simulink model "MoPhongRBKC"  (R2016a)
settings: Solver=VariableStepAuto  StartTime=0.0  StopTime=160  RelTol=1e-3
libraries: mblibv1 x18, simulink x3
settings Model: Creator=Nguyen Nam  LastModifiedBy=nguye
settings OptimizationCC: BlockReduction=off
settings GRTTargetCC: GeneratePreprocessorConditionals=Use local settings
settings SimMechanicsCC: VisOnUpdateDiagram=on  VisDuringSimulation=on

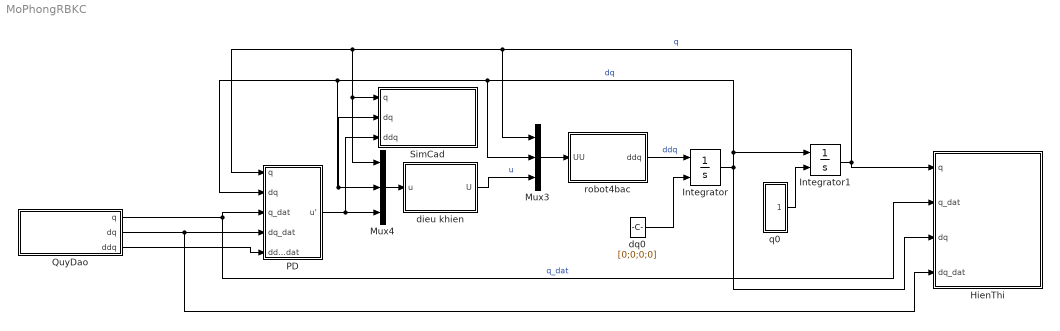
== system MoPhongRBKC ==
  HienThi : Subsystem  TreatAsAtomicUnit=on
  Integrator : Integrator  InitialConditionSource=external
  Integrator1 : Integrator  InitialConditionSource=external
  Mux3 : Mux  Inputs=3
  Mux4 : Mux  Inputs=3
  "PD " : Subsystem
  QuyDao : Subsystem  TreatAsAtomicUnit=on
  SimCad : Subsystem  TreatAsAtomicUnit=on
  dieu khien : MATLAB Function  TreatAsAtomicUnit=on
  dq0 : Constant  Value=[0;0;0;0]
  q0 : Subsystem
  robot4bac : MATLAB Function  TreatAsAtomicUnit=on
  wires:
  QuyDao/1(q) -> HienThi/2(q_dat), "PD "/3(q_dat)  "q_dat"
  Mux3/1 -> robot4bac/1(UU)
  robot4bac/1(ddq) -> Integrator/1  "ddq"
  Integrator/1 -> HienThi/3(dq), "PD "/2(dq), Mux4/2, SimCad/2(dq), Mux3/2, Integrator1/1  "dq"
  Integrator1/1 -> "PD "/1(q), Mux4/1, SimCad/1(q), Mux3/1, HienThi/1(q)  "q"
  q0/1("q0 ") -> Integrator1/2
  dq0/1 -> Integrator/2
  Mux4/1 -> dieu khien/1(u)
  "PD "/1(u') -> SimCad/3(ddq), Mux4/3
  dieu khien/1(U) -> Mux3/3  "u"
  QuyDao/3(ddq) -> "PD "/5(ddq_dat)
  QuyDao/2(dq) -> HienThi/4(dq_dat), "PD "/4(dq_dat)

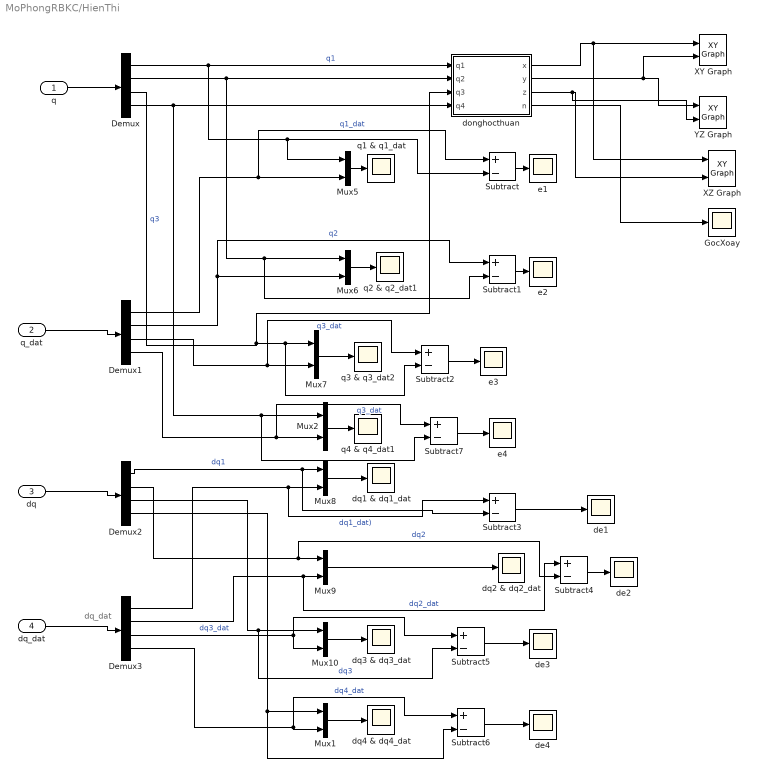
== system MoPhongRBKC/HienThi ==
  note: dq_dat
  q : Inport
  q_dat : Inport  Port=2
  dq : Inport  Port=3
  dq_dat : Inport  Port=4
  Demux{,1..3} (4 alike) : Demux
  GocXoay : Scope
  Mux{1..2,5..10} (8 alike) : Mux  Inputs=2
  Subtract{,1..7} (8 alike) : Sum  Inputs=+-
  XY Graph : simulink/Sinks/XY Graph  xmin=-10  xmax=500  ymin=-10  ymax=300  st=0
  XZ Graph : simulink/Sinks/XY Graph  xmin=-100  xmax=500  ymin=-100  ymax=300  st=0
  YZ Graph : simulink/Sinks/XY Graph  xmin=-100  xmax=300  ymin=-100  ymax=300  st=0
  de{1..4} (4 alike) : Scope
  donghocthuan : MATLAB Function  TreatAsAtomicUnit=on
  dq1 & dq1_dat : Scope
  dq2 & dq2_dat : Scope
  dq3 & dq3_dat : Scope
  dq4 & dq4_dat : Scope
  e{1..4} (4 alike) : Scope
  q1 & q1_dat : Scope
  q2 & q2_dat1 : Scope
  q3 & q3_dat2 : Scope
  q4 & q4_dat1 : Scope
  wires:
  q/1 -> Demux/1
  Demux/1 -> Subtract/2, Mux5/1, donghocthuan/1(q1)  "q1"
  Mux5/1 -> q1 & q1_dat/1
  Demux/2 -> Subtract1/2, Mux6/1, donghocthuan/2(q2)
  Demux1/2 -> Mux6/2, Subtract1/1  "q2"
  Demux1/3 -> Subtract2/1, Mux7/2  "q3_dat"
  Mux6/1 -> q2 & q2_dat1/1
  Demux2/1 -> Subtract3/2, Mux8/1  "dq1"
  Demux3/1 -> Subtract3/1, Mux8/2  "dq1_dat)"
  Mux8/1 -> dq1 & dq1_dat/1
  Demux2/2 -> Subtract4/2, Mux9/1  "dq2"
  Demux3/2 -> Subtract4/1, Mux9/2  "dq2_dat"
  Demux3/3 -> Mux10/2, Subtract5/1  "dq3_dat"
  Demux2/3 -> Subtract5/2, Mux10/1  "dq3"
  Mux10/1 -> dq3 & dq3_dat/1
  Mux9/1 -> dq2 & dq2_dat/1
  Mux7/1 -> q3 & q3_dat2/1
  Demux1/1 -> Subtract/1, Mux5/2  "q1_dat"
  donghocthuan/1(x) -> XZ Graph/1, XY Graph/1
  donghocthuan/2(y) -> YZ Graph/1, XY Graph/2
  Subtract/1 -> e1/1
  Subtract1/1 -> e2/1
  Subtract2/1 -> e3/1
  Subtract3/1 -> de1/1
  Subtract4/1 -> de2/1
  Subtract5/1 -> de3/1
  q_dat/1 -> Demux1/1
  dq/1 -> Demux2/1
  dq_dat/1 -> Demux3/1
  donghocthuan/4(n) -> GocXoay/1
  Demux/4 -> Subtract7/2, Mux2/1, donghocthuan/4(q4)
  Demux3/4 -> Mux1/2, Subtract6/1  "dq4_dat"
  Demux2/4 -> Subtract6/2, Mux1/1
  Mux1/1 -> dq4 & dq4_dat/1
  Subtract6/1 -> de4/1
  Demux1/4 -> Subtract7/1, Mux2/2  "q3_dat"
  Demux/3 -> donghocthuan/3(q3), Subtract2/2, Mux7/1  "q3"
  Mux2/1 -> q4 & q4_dat1/1
  Subtract7/1 -> e4/1
  donghocthuan/3(z) -> YZ Graph/2, XZ Graph/2

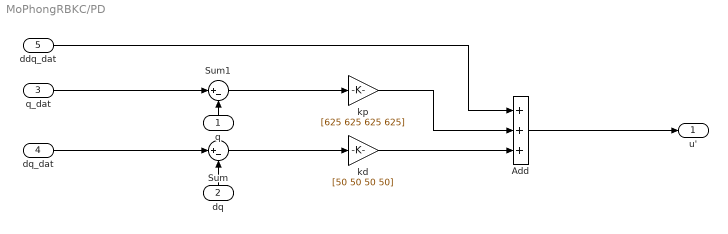
== system MoPhongRBKC/PD  ==
  q : Inport
  dq : Inport  Port=2
  q_dat : Inport  Port=3
  dq_dat : Inport  Port=4
  ddq_dat : Inport  Port=5
  Add : Sum  Inputs=3
  Sum : Sum  Inputs=|+-
  Sum1 : Sum  Inputs=|+-
  kd : Gain  Gain=[50 50 50 50]
  kp : Gain  Gain=[625 625 625 625]
  u' : Outport
  wires:
  Sum1/1 -> kp/1
  Sum/1 -> kd/1
  Add/1 -> u'/1
  ddq_dat/1 -> Add/1
  dq_dat/1 -> Sum/1
  q_dat/1 -> Sum1/1
  dq/1 -> Sum/2
  q/1 -> Sum1/2
  kd/1 -> Add/3
  kp/1 -> Add/2

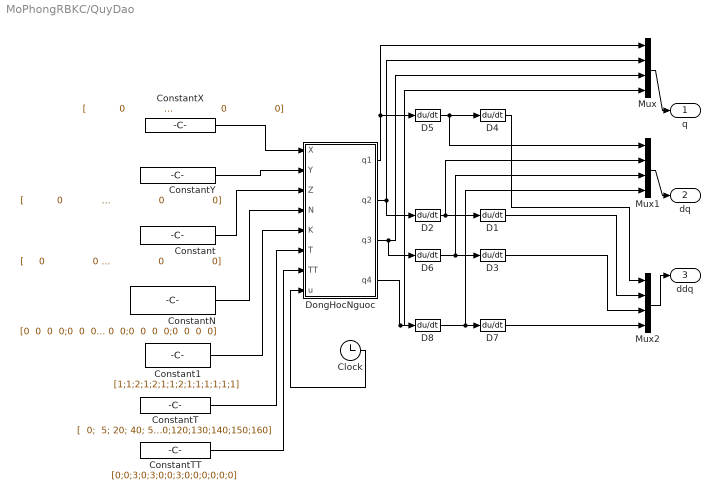
== system MoPhongRBKC/QuyDao ==
  Clock : Clock
      settings: Decimation=600
  Constant : Constant  Value="[     0                0               -6              0.8                0                0;   -50                0                0                0                0                0;   -50                0                0                0              -50                0;   -50                0                0                0                0                0;   -50                0                0                0              -50                0;   -50                0                0                0                0                0;   -50                0                0                0                0                0;   -50                0                0                0              -50                0;   -50                0                0                0                0                0;   -50                0                0                0                0                0;   -50                0                0                0                0                0;   -50                0                0                0                0                0;   -50                0                0                0                0                0;371200            -7200             46.5             -0.1                0                0]"
  Constant1 : Constant  Value=[1;1;2;1;2;1;1;2;1;1;1;1;1;1]
  ConstantN : Constant  Value="[0  0  0  0;0  0  0  0;0  0  0  0;0  0  0  0;0  0  0  0;0  0  0  0;0  0  0  0;0  0  0  0;0  0  0  0;0  0  0  0;0  0  0  0;0  0  0  0;0  0  0  0;0  0  0  0]"
  ConstantT : Constant  Value="[  0;  5; 20; 40; 50; 70; 80; 90;100;110;120;130;140;150;160]"
  ConstantTT : Constant  Value=[0;0;3;0;3;0;0;3;0;0;0;0;0;0]
  ConstantX : Constant  Value="[           0                0                0                0                0                0; 15.27777778     -6.666666667     0.8333333333   -0.02222222222                0                0; 14.13716694     -1.884955592    0.07068583471 -0.0007853981634               75             37.5;     31792.5            -2160             48.6            -0.36                0                0; 155.5088364     -8.246680716     0.1413716694 -0.0007853981634              330             37.5;       27440            -1092           14.625           -0.065                0                0;         400                0                0                0                0                0;-2670.353756      84.82300165    -0.8953539063   0.003141592654              390               10;     -229610             6600              -63              0.2                0                0;      -90460             2376            -20.7             0.06                0                0;     -621820            14976             -120             0.32                0                0;     -490000            10920              -81              0.2                0                0;           0                0                0                0                0                0;           0                0                0                0                0                0]"
  ConstantY : Constant  Value="[           0                0                0                0                0                0;           0                0                0                0                0                0; 14.13716694     -1.884955592    0.07068583471 -0.0007853981634                0             37.5;           0                0                0                0                0                0; 155.5088364     -8.246680716     0.1413716694 -0.0007853981634                0             37.5;           0                0                0                0                0                0;       85120            -3024             35.7            -0.14                0                0;-2670.353756      84.82300165    -0.8953539063   0.003141592654               70               10;          80                0                0                0                0                0;      121080            -3168             27.6            -0.08                0                0;         120                0                0                0                0                0;     -269435             6006           -44.55             0.11                0                0;     -394875             8190           -56.55             0.13                0                0;           0                0                0                0                0                0]"
  D{1..8} (8 alike) : Derivative
  DongHocNguoc : MATLAB Function  TreatAsAtomicUnit=on
  Mux : Mux
  Mux1 : Mux
  Mux2 : Mux
  q : Outport
  dq : Outport  Port=2
  ddq : Outport  Port=3
  wires:
  ConstantT/1 -> DongHocNguoc/6(T)
  ConstantY/1 -> DongHocNguoc/2(Y)
  ConstantX/1 -> DongHocNguoc/1(X)
  Constant/1 -> DongHocNguoc/3(Z)
  Constant1/1 -> DongHocNguoc/5(K)
  DongHocNguoc/1(q1) -> Mux/1, D5/1
  D5/1 -> Mux1/1, D4/1
  Clock/1 -> DongHocNguoc/8(u)
  ConstantN/1 -> DongHocNguoc/4(N)
  Mux/1 -> q/1
  DongHocNguoc/2(q2) -> D2/1, Mux/2
  DongHocNguoc/3(q3) -> D6/1, Mux/3
  DongHocNguoc/4(q4) -> D8/1, Mux/4
  Mux1/1 -> dq/1
  D2/1 -> Mux1/2, D1/1
  D6/1 -> Mux1/3, D3/1
  D8/1 -> Mux1/4, D7/1
  Mux2/1 -> ddq/1
  D4/1 -> Mux2/1
  D1/1 -> Mux2/2
  D3/1 -> Mux2/3
  D7/1 -> Mux2/4
  ConstantTT/1 -> DongHocNguoc/7(TT)

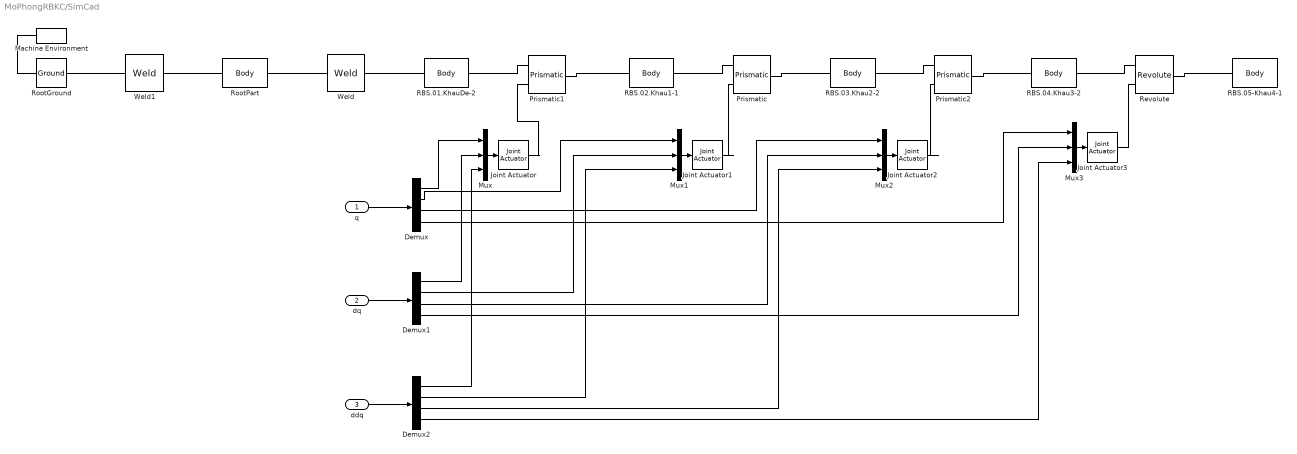
== system MoPhongRBKC/SimCad ==
  q : Inport
  dq : Inport  Port=2
  ddq : Inport  Port=3
  Demux : Demux
  Demux1 : Demux
  Demux2 : Demux
  Joint Actuator : mblibv1/Sensors &  Actuators/Joint Actuator  UpdateFromCAD=off  PhysicalDomain=Mechanical  PortType=blob  ActuationStyle=Motion  AngleUnits=deg  ArcVelocityUnits=deg/s  ArcAccelerationUnits=deg/s^2  CoordPositionUnits=mm  VelocityUnits=mm/s  AccelerationUnits=mm/s^2  ForceUnits=mN  TorqueUnits=N*m  ActiveIO=on  Width=3  DialogClass=MechanicalActuatorBlock  Primitive=P1  ReferenceFrame=Absolute (World)
  Joint Actuator1 : mblibv1/Sensors &  Actuators/Joint Actuator  UpdateFromCAD=off  PhysicalDomain=Mechanical  PortType=blob  ActuationStyle=Motion  AngleUnits=deg  ArcVelocityUnits=deg/s  ArcAccelerationUnits=deg/s^2  CoordPositionUnits=mm  VelocityUnits=mm/s  AccelerationUnits=mm/s^2  ForceUnits=mN  TorqueUnits=N*m  ActiveIO=on  Width=3  DialogClass=MechanicalActuatorBlock  Primitive=P1  ReferenceFrame=Absolute (World)
  Joint Actuator2 : mblibv1/Sensors &  Actuators/Joint Actuator  UpdateFromCAD=off  PhysicalDomain=Mechanical  PortType=blob  ActuationStyle=Motion  AngleUnits=deg  ArcVelocityUnits=deg/s  ArcAccelerationUnits=deg/s^2  CoordPositionUnits=mm  VelocityUnits=mm/s  AccelerationUnits=mm/s^2  ForceUnits=mN  TorqueUnits=N*m  ActiveIO=on  Width=3  DialogClass=MechanicalActuatorBlock  Primitive=P1  ReferenceFrame=Absolute (World)
  Joint Actuator3 : mblibv1/Sensors &  Actuators/Joint Actuator  UpdateFromCAD=off  PhysicalDomain=Mechanical  PortType=blob  ActuationStyle=Motion  AngleUnits=rad  ArcVelocityUnits=rad/s  ArcAccelerationUnits=rad/s^2  CoordPositionUnits=m  VelocityUnits=m/s  AccelerationUnits=m/s^2  ForceUnits=mN  TorqueUnits=N*m  ActiveIO=on  Width=3  DialogClass=MechanicalActuatorBlock  Primitive=R1  ReferenceFrame=Absolute (World)
  Machine Environment : mblibv1/Bodies/Machine Environment  PortType=env  PhysicalDomain=Mechanical  DialogTemplateClass=MECH.MachineEnvironment  SyncWhenCopied=off  Gravity=[0 -9.81 0]  GravityUnits=m/s^2  GravityAsSignal=off  Dimensionality=Auto-detect  AnalysisType=Forward dynamics  LinearAssemblyTolerance=1e-3  LinearAssemblyToleranceUnits=m  AngularAssemblyTolerance=1e-3  AngularAssemblyToleranceUnits=rad  ConstraintSolverType=Stabilizing  ConstraintRelTolerance=1e-4  ConstraintAbsTolerance=1e-4  UseRobustSingularityHandling=off  RedundancyAnalysisToleranceType=Automatically select tolerance  RedundancyAnalysisTolerance=1e-14  StatePerturbationType=Fixed  PerturbationSize=1e-5  VisualizeMachine=on  BodyVisualizationType=Use model default body geometries  BodyColorSelMode=Use model default  DefaultBodyColor=[1 0 0]
  Mux{,1..3} (4 alike) : Mux  Inputs=3
  Prismatic : mblibv1/Joints/Prismatic  LConnTagsString=__newl0|SA1  RConnTagsString=__newr0  UpdateFromCAD=on  NumSAPorts=1  CutJoint=off  MarkAsCut=off  Primitives=prismatic  PrimitiveProps=P1$World$[-1,0,0]$prismatic  DialogClass=JointBlock  P1Axis=[-1,0,0]
  Prismatic1 : mblibv1/Joints/Prismatic  LConnTagsString=__newl0|SA1  RConnTagsString=__newr0  UpdateFromCAD=on  NumSAPorts=1  CutJoint=off  MarkAsCut=off  Primitives=prismatic  PrimitiveProps=P1$World$[0,0,1]$prismatic  DialogClass=JointBlock  P1Axis=[0,0,1]
  Prismatic2 : mblibv1/Joints/Prismatic  LConnTagsString=__newl0|SA1  RConnTagsString=__newr0  UpdateFromCAD=on  NumSAPorts=1  CutJoint=off  MarkAsCut=off  Primitives=prismatic  PrimitiveProps=P1$World$[0,-1,0]$prismatic  DialogClass=JointBlock  P1Axis=[0,-1,0]
  RBS.01.KhauDe-2 : mblibv1/Bodies/Body  LConnTagsString=CS2  RConnTagsString=CS3  UpdateFromCAD=on  DialogClass=MechanicalBodyBlock  Mass=0.481266  MassUnits=kg  InertiaUnits=kg*m^2  Inertia=[3.26313,0,0;0,3.76071,0;0,0,1.18222]  Shape=Cylinder  ShapeDims=[1 1]  ShapeUnits=m  ShapeUse=false  Density=1  DensityUnits=kg/m^3  DensityUse=false  GraphicsMode=GFXFILE  GraphicsFileName=sualai - RBS.01.KhauDe-2.STL  BodyColorSelMode=COLORPALETTE  BodyColor=[0.65098;0.619608;0.588235]  AttachedToCS=CS1  CG=Right$CG$[1.35 0.730871 2.35]$WORLD$WORLD$m$[1 0 0;0 1 0;0 0 1]$3x3 Transform$rad$WORLD$false$none  WorkingFrames=Right$CS1$[0 0 0]$WORLD$WORLD$m$[1 0 0;0 1 0;0 0 1]$3x3 Transform$rad$WORLD$false$none#Left$CS2$[1.35 0.730871 2.35]$WORLD$WORLD$m$[1 0 0;0 1 0;0 0 1]$3x3 Transform$rad$WORLD$true$none#Right$CS3$[0.283311 0.05 2.89491]$WORLD$WORLD$m$[1 0 0;0 1 0;0 0 1]$3x3 Transform$rad$WORLD$true$none  CGPos=[1.35 0.730871 2.35]  CGRot=[1 0 0;0 1 0;0 0 1]  CS0Pos=[]  CS0Rot=[]  CS1Pos=[0 0 0]  CS1Rot=[1 0 0;0 1 0;0 0 1]  CS2Pos=[1.35 0.730871 2.35]  CS2Rot=[1 0 0;0 1 0;0 0 1]  CS3Pos=[0.283311 0.05 2.89491]  CS3Rot=[1 0 0;0 1 0;0 0 1]  CS4Pos=[]  CS4Rot=[]  CS5Pos=[]  CS5Rot=[]  CS6Pos=[]  CS6Rot=[]  CS7Pos=[]  CS7Rot=[]  CS8Pos=[]  CS8Rot=[]  CS9Pos=[]  CS9Rot=[]  CS10Pos=[]  CS10Rot=[]  CS11Pos=[]  CS11Rot=[]  CS12Pos=[]  CS12Rot=[]  CS13Pos=[]  CS13Rot=[]  CS14Pos=[]  CS14Rot=[]  CS15Pos=[]  CS15Rot=[]  CS16Pos=[]  CS16Rot=[]  CS17Pos=[]  CS17Rot=[]  CS18Pos=[]  CS18Rot=[]  CS19Pos=[]  CS19Rot=[]  CS20Pos=[]  CS20Rot=[]
  RBS.02.Khau1-1 : mblibv1/Bodies/Body  LConnTagsString=CS3  RConnTagsString=CS2  UpdateFromCAD=on  DialogClass=MechanicalBodyBlock  Mass=0.091  MassUnits=kg  InertiaUnits=kg*m^2  Inertia=[0.0767067,0,0;0,0.0683701,0;0,0,0.00850512]  Shape=Cylinder  ShapeDims=[1 1]  ShapeUnits=m  ShapeUse=false  Density=1  DensityUnits=kg/m^3  DensityUse=false  GraphicsMode=GFXFILE  GraphicsFileName=sualai - RBS.02.Khau1-1.STL  BodyColorSelMode=COLORPALETTE  BodyColor=[0.65098;0.619608;0.588235]  AttachedToCS=CS1  CG=Right$CG$[1.35 -0.0387363 1.523]$WORLD$WORLD$m$[0 0 1;-1 0 0;0 -1 0]$3x3 Transform$rad$WORLD$false$none  WorkingFrames=Right$CS1$[0.2 -0.1 1.523]$WORLD$WORLD$m$[0 0 1;-1 0 0;0 -1 0]$3x3 Transform$rad$WORLD$false$none#Right$CS2$[0.44375 -0.1 1.35269]$WORLD$WORLD$m$[1 0 0;0 1 0;0 0 1]$3x3 Transform$rad$WORLD$true$none#Left$CS3$[0.283311 0.05 2.89491]$WORLD$WORLD$m$[1 0 0;0 1 0;0 0 1]$3x3 Transform$rad$WORLD$true$none  CGPos=[1.35 -0.0387363 1.523]  CGRot=[0 0 1;-1 0 0;0 -1 0]  CS0Pos=[]  CS0Rot=[]  CS1Pos=[0.2 -0.1 1.523]  CS1Rot=[0 0 1;-1 0 0;0 -1 0]  CS2Pos=[0.44375 -0.1 1.35269]  CS2Rot=[1 0 0;0 1 0;0 0 1]  CS3Pos=[0.283311 0.05 2.89491]  CS3Rot=[1 0 0;0 1 0;0 0 1]  CS4Pos=[]  CS4Rot=[]  CS5Pos=[]  CS5Rot=[]  CS6Pos=[]  CS6Rot=[]  CS7Pos=[]  CS7Rot=[]  CS8Pos=[]  CS8Rot=[]  CS9Pos=[]  CS9Rot=[]  CS10Pos=[]  CS10Rot=[]  CS11Pos=[]  CS11Rot=[]  CS12Pos=[]  CS12Rot=[]  CS13Pos=[]  CS13Rot=[]  CS14Pos=[]  CS14Rot=[]  CS15Pos=[]  CS15Rot=[]  CS16Pos=[]  CS16Rot=[]  CS17Pos=[]  CS17Rot=[]  CS18Pos=[]  CS18Rot=[]  CS19Pos=[]  CS19Rot=[]  CS20Pos=[]  CS20Rot=[]
  RBS.03.Khau2-2 : mblibv1/Bodies/Body  LConnTagsString=CS2  RConnTagsString=CS3  UpdateFromCAD=on  DialogClass=MechanicalBodyBlock  Mass=678.24  MassUnits=kg  InertiaUnits=kg*m^2  Inertia=[193.644,0,0;0,196.51,-6.39404;0,-6.39404,12.4099]  Shape=Cylinder  ShapeDims=[1 1]  ShapeUnits=m  ShapeUse=false  Density=1  DensityUnits=kg/m^3  DensityUse=false  GraphicsMode=GFXFILE  GraphicsFileName=sualai - RBS.03.Khau2-2.STL  BodyColorSelMode=COLORPALETTE  BodyColor=[1;0;0]  AttachedToCS=CS1  CG=Right$CG$[0.623217 -0.135278 1.523]$WORLD$WORLD$m$[0 1 0;0 0 1;1 0 0]$3x3 Transform$rad$WORLD$false$none  WorkingFrames=Right$CS1$[0.809559 -1.09 1.523]$WORLD$WORLD$m$[0 1 0;0 0 1;1 0 0]$3x3 Transform$rad$WORLD$false$none#Left$CS2$[0.44375 -0.1 1.35269]$WORLD$WORLD$m$[1 0 0;0 1 0;0 0 1]$3x3 Transform$rad$WORLD$true$none#Right$CS3$[0.709559 -0.75 1.423]$WORLD$WORLD$m$[1 0 0;0 1 0;0 0 1]$3x3 Transform$rad$WORLD$true$none  CGPos=[0.623217 -0.135278 1.523]  CGRot=[0 1 0;0 0 1;1 0 0]  CS0Pos=[]  CS0Rot=[]  CS1Pos=[0.809559 -1.09 1.523]  CS1Rot=[0 1 0;0 0 1;1 0 0]  CS2Pos=[0.44375 -0.1 1.35269]  CS2Rot=[1 0 0;0 1 0;0 0 1]  CS3Pos=[0.709559 -0.75 1.423]  CS3Rot=[1 0 0;0 1 0;0 0 1]  CS4Pos=[]  CS4Rot=[]  CS5Pos=[]  CS5Rot=[]  CS6Pos=[]  CS6Rot=[]  CS7Pos=[]  CS7Rot=[]  CS8Pos=[]  CS8Rot=[]  CS9Pos=[]  CS9Rot=[]  CS10Pos=[]  CS10Rot=[]  CS11Pos=[]  CS11Rot=[]  CS12Pos=[]  CS12Rot=[]  CS13Pos=[]  CS13Rot=[]  CS14Pos=[]  CS14Rot=[]  CS15Pos=[]  CS15Rot=[]  CS16Pos=[]  CS16Rot=[]  CS17Pos=[]  CS17Rot=[]  CS18Pos=[]  CS18Rot=[]  CS19Pos=[]  CS19Rot=[]  CS20Pos=[]  CS20Rot=[]
  RBS.04.Khau3-2 : mblibv1/Bodies/Body  LConnTagsString=CS2  RConnTagsString=CS3  UpdateFromCAD=on  DialogClass=MechanicalBodyBlock  Mass=363.732  MassUnits=kg  InertiaUnits=kg*m^2  Inertia=[108.563,0,0;0,108.563,0;0,0,3.30044]  Shape=Cylinder  ShapeDims=[1 1]  ShapeUnits=m  ShapeUse=false  Density=1  DensityUnits=kg/m^3  DensityUse=false  GraphicsMode=GFXFILE  GraphicsFileName=sualai - RBS.04.Khau3-2.STL  BodyColorSelMode=COLORPALETTE  BodyColor=[0;1;1]  AttachedToCS=CS1  CG=Right$CG$[0.809559 1.1517 1.523]$WORLD$WORLD$m$[0 1 0;0 0 1;1 0 0]$3x3 Transform$rad$WORLD$false$none  WorkingFrames=Right$CS1$[0.809559 2.0111 1.523]$WORLD$WORLD$m$[0 1 0;0 0 1;1 0 0]$3x3 Transform$rad$WORLD$false$none#Left$CS2$[0.709559 -0.75 1.423]$WORLD$WORLD$m$[1 0 0;0 1 0;0 0 1]$3x3 Transform$rad$WORLD$true$none#Right$CS3$[0.809559 2.0111 1.523]$WORLD$WORLD$m$[1 0 0;0 1 0;0 0 1]$3x3 Transform$rad$WORLD$true$none  CGPos=[0.809559 1.1517 1.523]  CGRot=[0 1 0;0 0 1;1 0 0]  CS0Pos=[]  CS0Rot=[]  CS1Pos=[0.809559 2.0111 1.523]  CS1Rot=[0 1 0;0 0 1;1 0 0]  CS2Pos=[0.709559 -0.75 1.423]  CS2Rot=[1 0 0;0 1 0;0 0 1]  CS3Pos=[0.809559 2.0111 1.523]  CS3Rot=[1 0 0;0 1 0;0 0 1]  CS4Pos=[]  CS4Rot=[]  CS5Pos=[]  CS5Rot=[]  CS6Pos=[]  CS6Rot=[]  CS7Pos=[]  CS7Rot=[]  CS8Pos=[]  CS8Rot=[]  CS9Pos=[]  CS9Rot=[]  CS10Pos=[]  CS10Rot=[]  CS11Pos=[]  CS11Rot=[]  CS12Pos=[]  CS12Rot=[]  CS13Pos=[]  CS13Rot=[]  CS14Pos=[]  CS14Rot=[]  CS15Pos=[]  CS15Rot=[]  CS16Pos=[]  CS16Rot=[]  CS17Pos=[]  CS17Rot=[]  CS18Pos=[]  CS18Rot=[]  CS19Pos=[]  CS19Rot=[]  CS20Pos=[]  CS20Rot=[]
  RBS.05-Khau4-1 : mblibv1/Bodies/Body  LConnTagsString=CS2  UpdateFromCAD=on  DialogClass=MechanicalBodyBlock  Mass=26.144  MassUnits=kg  InertiaUnits=kg*m^2  Inertia=[0.122087,0,0;0,0.139242,0;0,0,0.219027]  Shape=Cylinder  ShapeDims=[1 1]  ShapeUnits=m  ShapeUse=false  Density=1  DensityUnits=kg/m^3  DensityUse=false  GraphicsMode=GFXFILE  GraphicsFileName=sualai - RBS.05-Khau4-1.STL  BodyColorSelMode=COLORPALETTE  BodyColor=[1;1;0]  AttachedToCS=CS1  CG=Right$CG$[0.809498 2.0611 1.52775]$WORLD$WORLD$m$[-0.0129085 0.999917 0;0 0 1;0.999917 0.0129085 0]$3x3 Transform$rad$WORLD$false$none  WorkingFrames=Right$CS1$[0.806332 2.0611 1.77298]$WORLD$WORLD$m$[-0.0129085 0.999917 0;0 0 1;0.999917 0.0129085 0]$3x3 Transform$rad$WORLD$false$none#Left$CS2$[0.809559 2.0111 1.523]$WORLD$WORLD$m$[1 0 0;0 1 0;0 0 1]$3x3 Transform$rad$WORLD$true$none  CGPos=[0.809498 2.0611 1.52775]  CGRot=[-0.0129085 0.999917 0;0 0 1;0.999917 0.0129085 0]  CS0Pos=[]  CS0Rot=[]  CS1Pos=[0.806332 2.0611 1.77298]  CS1Rot=[-0.0129085 0.999917 0;0 0 1;0.999917 0.0129085 0]  CS2Pos=[0.809559 2.0111 1.523]  CS2Rot=[1 0 0;0 1 0;0 0 1]  CS3Pos=[]  CS3Rot=[]  CS4Pos=[]  CS4Rot=[]  CS5Pos=[]  CS5Rot=[]  CS6Pos=[]  CS6Rot=[]  CS7Pos=[]  CS7Rot=[]  CS8Pos=[]  CS8Rot=[]  CS9Pos=[]  CS9Rot=[]  CS10Pos=[]  CS10Rot=[]  CS11Pos=[]  CS11Rot=[]  CS12Pos=[]  CS12Rot=[]  CS13Pos=[]  CS13Rot=[]  CS14Pos=[]  CS14Rot=[]  CS15Pos=[]  CS15Rot=[]  CS16Pos=[]  CS16Rot=[]  CS17Pos=[]  CS17Rot=[]  CS18Pos=[]  CS18Rot=[]  CS19Pos=[]  CS19Rot=[]  CS20Pos=[]  CS20Rot=[]
  Revolute : mblibv1/Joints/Revolute  LConnTagsString=__newl0|SA1  RConnTagsString=__newr0  UpdateFromCAD=on  NumSAPorts=1  CutJoint=off  MarkAsCut=off  Primitives=prismatic  PrimitiveProps=R1$World$[0,1,0]$revolute  DialogClass=JointBlock  R1Axis=[0,1,0]
  RootGround : mblibv1/Bodies/Ground  UpdateFromCAD=on  LeftPortType=env  RightPortType=workingframe  PhysicalDomain=Mechanical  DialogClass=GroundBlock  CoordPosition=[1.22346,0.560132,2.08492]  CoordPositionUnits=m  StateVectorMgrId=2  MachineId=[3 0]  ShowEnvPort=on  ParameterChecksum=[26115674, 4278191838, 2529439133, 1681005142]  TopologyChecksum=[1353211491, 567135128, 1435651920, 3166930891]
  RootPart : mblibv1/Bodies/Body  LConnTagsString=CS3  RConnTagsString=CS2  UpdateFromCAD=on  DialogClass=MechanicalBodyBlock  Mass=0  MassUnits=kg  InertiaUnits=kg*m^2  Inertia=[0,0,0;0,0,0;0,0,0]  Shape=Cylinder  ShapeDims=[1 1]  ShapeUnits=m  ShapeUse=false  Density=1  DensityUnits=kg/m^3  DensityUse=false  GraphicsMode=MACHINE_DEFAULT  BodyColorSelMode=MACHINE_DEFAULT  BodyColor=[1;0;0]  AttachedToCS=CS1  CG=Right$CG$[1.22346 0.560132 2.08492]$WORLD$WORLD$m$[1 0 0;0 1 0;0 0 1]$3x3 Transform$rad$WORLD$false$none  WorkingFrames=Right$CS1$[0 0 0]$WORLD$WORLD$m$[1 0 0;0 1 0;0 0 1]$3x3 Transform$rad$WORLD$false$none#Right$CS2$[1.35 0.730871 2.35]$WORLD$WORLD$m$[1 0 0;0 1 0;0 0 1]$3x3 Transform$rad$WORLD$true$none#Left$CS3$[1.22346 0.560132 2.08492]$WORLD$WORLD$m$[1 0 0;0 1 0;0 0 1]$3x3 Transform$rad$WORLD$true$none  CGPos=[1.22346 0.560132 2.08492]  CGRot=[1 0 0;0 1 0;0 0 1]  CS0Pos=[]  CS0Rot=[]  CS1Pos=[0 0 0]  CS1Rot=[1 0 0;0 1 0;0 0 1]  CS2Pos=[1.35 0.730871 2.35]  CS2Rot=[1 0 0;0 1 0;0 0 1]  CS3Pos=[1.22346 0.560132 2.08492]  CS3Rot=[1 0 0;0 1 0;0 0 1]  CS4Pos=[]  CS4Rot=[]  CS5Pos=[]  CS5Rot=[]  CS6Pos=[]  CS6Rot=[]  CS7Pos=[]  CS7Rot=[]  CS8Pos=[]  CS8Rot=[]  CS9Pos=[]  CS9Rot=[]  CS10Pos=[]  CS10Rot=[]  CS11Pos=[]  CS11Rot=[]  CS12Pos=[]  CS12Rot=[]  CS13Pos=[]  CS13Rot=[]  CS14Pos=[]  CS14Rot=[]  CS15Pos=[]  CS15Rot=[]  CS16Pos=[]  CS16Rot=[]  CS17Pos=[]  CS17Rot=[]  CS18Pos=[]  CS18Rot=[]  CS19Pos=[]  CS19Rot=[]  CS20Pos=[]  CS20Rot=[]
  Weld : mblibv1/Joints/Weld  LConnTagsString=__newl0  RConnTagsString=__newr0  UpdateFromCAD=on  NumSAPorts=0  CutJoint=off  MarkAsCut=off  Primitives=weld  PrimitiveProps=W$WORLD$[0.57735,0.57735,0.57735]$weld  DialogClass=JointBlock  WAxis=[0.57735,0.57735,0.57735]
  Weld1 : mblibv1/Joints/Weld  LConnTagsString=__newl0  RConnTagsString=__newr0  UpdateFromCAD=on  NumSAPorts=0  CutJoint=off  MarkAsCut=off  Primitives=weld  PrimitiveProps=W$WORLD$[0.57735,0.57735,0.57735]$weld  DialogClass=JointBlock  WAxis=[0.57735,0.57735,0.57735]
  wires:
  q/1 -> Demux/1
  dq/1 -> Demux1/1
  ddq/1 -> Demux2/1
  Mux/1 -> Joint Actuator/1
  Demux/1 -> Mux/1
  Demux1/1 -> Mux/2
  Demux2/1 -> Mux/3
  Mux1/1 -> Joint Actuator1/1
  Mux2/1 -> Joint Actuator2/1
  Mux3/1 -> Joint Actuator3/1
  Demux/2 -> Mux1/1
  Demux1/2 -> Mux1/2
  Demux2/2 -> Mux1/3
  Demux/3 -> Mux2/1
  Demux1/3 -> Mux2/2
  Demux2/3 -> Mux2/3
  Demux/4 -> Mux3/1
  Demux1/4 -> Mux3/2
  Demux2/4 -> Mux3/3
  connections:
  RBS.02.Khau1-1/RConn1 -- Prismatic/LConn1
  Prismatic/RConn1 -- RBS.03.Khau2-2/LConn1
  Weld/RConn1 -- RBS.01.KhauDe-2/LConn1
  RootGround/RConn1 -- Weld1/LConn1
  Prismatic1/RConn1 -- RBS.02.Khau1-1/LConn1
  Prismatic2/RConn1 -- RBS.04.Khau3-2/LConn1
  Weld1/RConn1 -- RootPart/LConn1
  RBS.03.Khau2-2/RConn1 -- Prismatic2/LConn1
  Revolute/RConn1 -- RBS.05-Khau4-1/LConn1
  RootGround/LConn1 -- Machine Environment/RConn1
  RBS.04.Khau3-2/RConn1 -- Revolute/LConn1
  RBS.01.KhauDe-2/RConn1 -- Prismatic1/LConn1
  RootPart/RConn1 -- Weld/LConn1
  Joint Actuator/RConn1 -- Prismatic1/LConn2
  Joint Actuator3/RConn1 -- Revolute/LConn2
  Joint Actuator2/RConn1 -- Prismatic2/LConn2
  Joint Actuator1/RConn1 -- Prismatic/LConn2

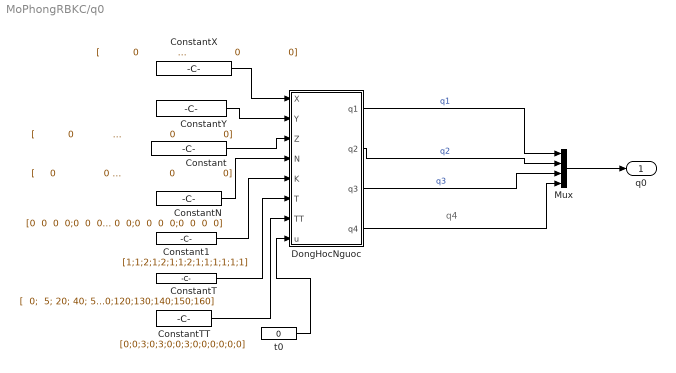
== system MoPhongRBKC/q0 ==
  note: q4
  Constant : Constant  Value="[     0                0               -6              0.8                0                0;   -50                0                0                0                0                0;   -50                0                0                0              -50                0;   -50                0                0                0                0                0;   -50                0                0                0              -50                0;   -50                0                0                0                0                0;   -50                0                0                0                0                0;   -50                0                0                0              -50                0;   -50                0                0                0                0                0;   -50                0                0                0                0                0;   -50                0                0                0                0                0;   -50                0                0                0                0                0;   -50                0                0                0                0                0;371200            -7200             46.5             -0.1                0                0]"
  Constant1 : Constant  Value=[1;1;2;1;2;1;1;2;1;1;1;1;1;1]
  ConstantN : Constant  Value="[0  0  0  0;0  0  0  0;0  0  0  0;0  0  0  0;0  0  0  0;0  0  0  0;0  0  0  0;0  0  0  0;0  0  0  0;0  0  0  0;0  0  0  0;0  0  0  0;0  0  0  0;0  0  0  0]"
  ConstantT : Constant  Value="[  0;  5; 20; 40; 50; 70; 80; 90;100;110;120;130;140;150;160]"
  ConstantTT : Constant  Value=[0;0;3;0;3;0;0;3;0;0;0;0;0;0]
  ConstantX : Constant  Value="[           0                0                0                0                0                0; 15.27777778     -6.666666667     0.8333333333   -0.02222222222                0                0; 14.13716694     -1.884955592    0.07068583471 -0.0007853981634               75             37.5;     31792.5            -2160             48.6            -0.36                0                0; 155.5088364     -8.246680716     0.1413716694 -0.0007853981634              330             37.5;       27440            -1092           14.625           -0.065                0                0;         400                0                0                0                0                0;-2670.353756      84.82300165    -0.8953539063   0.003141592654              390               10;     -229610             6600              -63              0.2                0                0;      -90460             2376            -20.7             0.06                0                0;     -621820            14976             -120             0.32                0                0;     -490000            10920              -81              0.2                0                0;           0                0                0                0                0                0;           0                0                0                0                0                0]"
  ConstantY : Constant  Value="[           0                0                0                0                0                0;           0                0                0                0                0                0; 14.13716694     -1.884955592    0.07068583471 -0.0007853981634                0             37.5;           0                0                0                0                0                0; 155.5088364     -8.246680716     0.1413716694 -0.0007853981634                0             37.5;           0                0                0                0                0                0;       85120            -3024             35.7            -0.14                0                0;-2670.353756      84.82300165    -0.8953539063   0.003141592654               70               10;          80                0                0                0                0                0;      121080            -3168             27.6            -0.08                0                0;         120                0                0                0                0                0;     -269435             6006           -44.55             0.11                0                0;     -394875             8190           -56.55             0.13                0                0;           0                0                0                0                0                0]"
  DongHocNguoc : MATLAB Function  TreatAsAtomicUnit=on
  Mux : Mux
  t0 : Constant  Value=0
  "q0 " : Outport
  wires:
  DongHocNguoc/1(q1) -> Mux/1  "q1"
  DongHocNguoc/2(q2) -> Mux/2  "q2"
  DongHocNguoc/3(q3) -> Mux/3  "q3"
  Mux/1 -> "q0 "/1
  ConstantT/1 -> DongHocNguoc/6(T)
  ConstantY/1 -> DongHocNguoc/2(Y)
  ConstantX/1 -> DongHocNguoc/1(X)
  Constant/1 -> DongHocNguoc/3(Z)
  Constant1/1 -> DongHocNguoc/5(K)
  t0/1 -> DongHocNguoc/8(u)
  ConstantN/1 -> DongHocNguoc/4(N)
  DongHocNguoc/4(q4) -> Mux/4
  ConstantTT/1 -> DongHocNguoc/7(TT)

== matlab function MoPhongRBKC/HienThi/donghocthuan ==
  data: q1 input; x output; q2 input; q3 input; y output; z output; q4 input; n output
function [x,y,z,n]=donghocthuan(q1,q2,q3,q4)
 x=q2 - 250*cos(q4);
 y=q3 - 50;
 z=q1 + 250*sin(q4);
 n=q4*180/pi;
 % Ve Do thi 3D 
%plot3(-z,y,x,'b.');
%hold on;
%grid on
% Bien Doi Toa do theo decac cho de nhin

== matlab function MoPhongRBKC/QuyDao/DongHocNguoc ==
  data: X input; Y input; Z input; N input; K input; T input; TT input; u input; q1 output; q2 output; q3 output; q4 output
function [q1,q2,q3,q4] = fcn(X,Y,Z,N,K,T,TT,u)
%#codegen
% X la ma tran n*6 hsx0 hsx1 hsx2 hsx3 Xi Bk
% Y la ma tran n*6 
% Z   //       n*6
% T la ma tran (n+1)*1 
% K la ma tran n*1 cot 1 DangChuyendong luon quay theo truc z
% u la bien chay thoi gian thuc
Ex=0;
Ey=0;
Ez=0;
Rz=0;
T=T;


for i=1:1:size(K,1)
    if (T(i,1) < u) && (u <= T(i+1))
        %kiem tra dang chuyen dong de gan he so
        if K(i,1) == 1 %chuyen dong thang
            Ex=X(i,1) + X(i,2)*u + X(i,3)*u*u + X(i,4)*u*u*u;
            Ey=Y(i,1) + Y(i,2)*u + Y(i,3)*u*u + Y(i,4)*u*u*u;
            Ez=Z(i,1) + Z(i,2)*u + Z(i,3)*u*u + Z(i,4)*u*u*u;
            Rz=0;
        end
        if K(i,1) == 2 %chuyen dong cung tron
            %kiem tra xem quay theo truc nao
            if TT(i,1)==3
            %Quay theo truc Z
                Ex=X(i,5) + X(i,6)*sin(X(i,1) + X(i,2)*u + X(i,3)*u*u + X(i,4)*u*u*u);
                Ey=Y(i,5) + Y(i,6)*cos(Y(i,1) + Y(i,2)*u + Y(i,3)*u*u + Y(i,4)*u*u*u);
                % neu X0==X1 thi
                %Ex=X(i,5) + X(i,6)*cos(X(i,1) + X(i,2)*u + X(i,3)*u*u + X(i,4)*u*u*u);
                %Ey=Y(i,5) + Y(i,6)*sin(Y(i,1) + Y(i,2)*u + Y(i,3)*u*u + Y(i,4)*u*u*u);
                Ez=Z(i,1) + Z(i,2)*u + Z(i,3)*u*u + Z(i,4)*u*u*u;
                Rz=0;
            end
            if TT(i,1)==2
            %Quay theo truc Y
                Ex=X(i,5) + X(i,6)*sin(X(i,1) + X(i,2)*u + X(i,3)*u*u + X(i,4)*u*u*u);
                Ey=Y(i,1) + Y(i,2)*u + Y(i,3)*u*u + Y(i,4)*u*u*u;
                Ez=Z(i,5) + Z(i,6)*cos(Z(i,1) + Z(i,2)*u + Z(i,3)*u*u + Z(i,4)*u*u*u);
                Rz=0;
                
            end
            if TT(i,1)==1
            %Quay theo truc X
                Ex=X(i,1) + X(i,2)*u + X(i,3)*u*u + X(i,4)*u*u*u;
                Ey=Y(i,5) + Y(i,6)*sin(Y(i,1) + Y(i,2)*u + Y(i,3)*u*u + Y(i,4)*u*u*u);
                Ez=Z(i,5) + Z(i,6)*cos(Z(i,1) + Z(i,2)*u + Z(i,3)*u*u + Z(i,4)*u*u*u);
                Rz=0;
                
            end
        end
        if K(i,1) == 3 % Chuyen dong quay rz q4
            Rz=N(i,1) + N(i,2)*u + N(i,3)*u*u + N(i,4)*u*u*u;
            Ex=0;
            Ey=0;
            Ez=0;
        end
    end
% Dong hoc nguoc
     
     q1=Ez - 250*sin(Rz);
     q2=Ex + 250*cos(Rz);
     q3=Ey + 50;
     q4=Rz;
end
end

== matlab function MoPhongRBKC/q0/DongHocNguoc ==
  data: X input; Y input; Z input; N input; K input; T input; TT input; u input; q1 output; q2 output; q3 output; q4 output
function [q1,q2,q3,q4] = fcn(X,Y,Z,N,K,T,TT,u)
%#codegen
% X la ma tran n*6 hsx0 hsx1 hsx2 hsx3 Xi Bk
% Y la ma tran n*6 
% Z   //       n*6
% T la ma tran (n+1)*1 
% K la ma tran n*1 cot 1 DangChuyendong luon quay theo truc z
% u la bien chay thoi gian thuc
Ex=0;
Ey=0;
Ez=0;
Rz=0;
T=T;

for i=1:1:size(K,1)
    if (T(i,1) < u) && (u <= T(i+1))
        %kiem tra dang chuyen dong de gan he so
        if K(i,1) == 1 %chuyen dong thang
            Ex=X(i,1) + X(i,2)*u + X(i,3)*u*u + X(i,4)*u*u*u;
            Ey=Y(i,1) + Y(i,2)*u + Y(i,3)*u*u + Y(i,4)*u*u*u;
            Ez=Z(i,1) + Z(i,2)*u + Z(i,3)*u*u + Z(i,4)*u*u*u;
            Rz=0;
        end
        if K(i,1) == 2 %chuyen dong cung tron
            %kiem tra xem quay theo truc nao
            if TT(i,1)==3
            %Quay theo truc Z
                Ex=X(i,5) + X(i,6)*sin(X(i,1) + X(i,2)*u + X(i,3)*u*u + X(i,4)*u*u*u);
                Ey=Y(i,5) + Y(i,6)*cos(Y(i,1) + Y(i,2)*u + Y(i,3)*u*u + Y(i,4)*u*u*u);
                Ez=Z(i,1) + Z(i,2)*u + Z(i,3)*u*u + Z(i,4)*u*u*u;
                Rz=0;
            end
            if TT(i,1)==2
            %Quay theo truc Y
                Ex=X(i,5) + X(i,6)*sin(X(i,1) + X(i,2)*u + X(i,3)*u*u + X(i,4)*u*u*u);
                Ey=Y(i,1) + Y(i,2)*u + Y(i,3)*u*u + Y(i,4)*u*u*u;
                Ez=Z(i,5) + Z(i,6)*cos(Z(i,1) + Z(i,2)*u + Z(i,3)*u*u + Z(i,4)*u*u*u);
                Rz=0;
                
            end
            if TT(i,1)==1
            %Quay theo truc X
                Ex=X(i,1) + X(i,2)*u + X(i,3)*u*u + X(i,4)*u*u*u;
                Ey=Y(i,5) + Y(i,6)*sin(Y(i,1) + Y(i,2)*u + Y(i,3)*u*u + Y(i,4)*u*u*u);
                Ez=Z(i,5) + Z(i,6)*cos(Z(i,1) + Z(i,2)*u + Z(i,3)*u*u + Z(i,4)*u*u*u);
                Rz=0;
                
            end
        end
        if K(i,1) == 3 % Chuyen dong quay rz q4
            Rz=N(i,1) + N(i,2)*u + N(i,3)*u*u + N(i,4)*u*u*u;
            Ex=0;
            Ey=0;
            Ez=0;
        end
    end
% Dong hoc nguoc
     
     q1=Ez - 250*sin(Rz);
     q2=Ex + 250*cos(Rz);
     q3=Ey + 50;
     q4=Rz;
end
end

== matlab function MoPhongRBKC/dieu khien ==
  data: u input; U output
function U=dieukhien(u)

% Thong cac bien dau vao
q=u(1:4);
q1=q(1);q2=q(2);q3=q(3);q4=q(4);
dq=u(5:8);
dq1=dq(1);dq2=dq(2);dq3=dq(3);dq4=dq(4);
ddq=u(9:12);
ddq1=ddq(1);ddq2=ddq(2);ddq3=ddq(3);ddq4=ddq(4)

%MA TRAN KHOI LUONG
Mqq =[                                                            (891233*ddq1)/500 + 6536*ddq4*cos(q4)
                                                                  (267029*ddq2)/250 + 6536*ddq4*sin(q4)
                                                                                       (97469*ddq3)/250
       ddq4*(1634000*cos(q4)^2 + 1634000*sin(q4)^2 + 122086897) + 6536*ddq1*cos(q4) + 6536*ddq2*sin(q4)];
%LUC QUAN TINH CORIOLIS
cqq =[-6536*dq4^2*sin(q4)
       6536*dq4^2*cos(q4)
                       0
                       0];
%MA TRAN G(q)
Gq =[                                0
                                     0
      -4511914398182529/17592186044416
                                     0];
%LUC SUY RONG KHONG THE
Q =[0
    0
    0
    0];
 
% Phuong trinh vi phan chuyen dong;
% luc va momen dieu khien U 4*1 U1 U2 U3 luc tinh tien U4 momen quay
U=Mqq+cqq+Gq+Q;

== matlab function MoPhongRBKC/robot4bac ==
  data: UU input; ddq output
function ddq=robot(UU)

% Thong so tinh toan
q=UU(1:4);
q1=q(1);q2=q(2);q3=q(3);q4=q(4);
dq=UU(5:8);
dq1=dq(1);dq2=dq(2);dq3=dq(3);dq4=dq(4);
U=[UU(9);UU(10);UU(11);UU(12)];
U1=U(1);U2=U(2);U3=U(3);U4=U(4);
%MA TRAN KHOI LUONG
Mq =[   891233/500,            0,         0,                                      6536*cos(q4)
                 0,   267029/250,         0,                                      6536*sin(q4)
                 0,            0, 97469/250,                                                 0
      6536*cos(q4), 6536*sin(q4),         0, 1634000*cos(q4)^2 + 1634000*sin(q4)^2 + 122086897];
 
%LUC QUAN TINH CORIOLIS
cqq =[-6536*dq4^2*sin(q4)
       6536*dq4^2*cos(q4)
                       0
                       0];
%MA TRAN G(q)
Gq =[                                0
                                     0
      -4511914398182529/17592186044416
                                     0];
%LUC SUY RONG KHONG THE
Q =[0
    0
    0
    0];
%PHUONG TRINH VI PHAN CHUYEN DONG
ddq=Mq\(U-cqq-Gq-Q);
